simulink model "BODE"  (R2018b)
settings: Solver=VariableStepAuto  StartTime=0.0  StopTime=10.0  RelTol=1e-3
libraries: slctrlblks x1
settings Model: Creator=xpess  LastModifiedBy=xpess

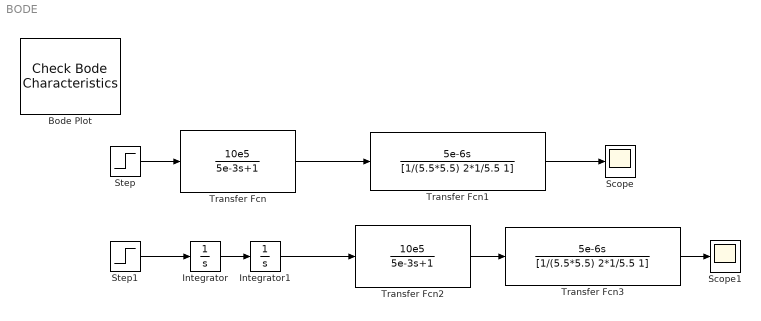
== system BODE ==
  Bode Plot : slctrlblks/Model Verification/Check Bode  Characteristics  InstantiateOnLoad=on  SaveOperatingPoints=off  LinearizationIOs={'/Step', 1, 'in', 'on', '';'/Transfer Fcn1', 1, 'out', 'on', ''}  LinearizeAt=SnapshotTimes  SnapshotTimes=[0]  TriggerType=rising  SampleTime=auto  RateConversionMethod=zoh  PreWarpFreq=10  UseExactDelayModel=off  UseFullBlockNameLabels=off  UseBusSignalLabels=off  enabled=on  stopWhenAssertionFail=off  export=off  ViewDlgPos=[412.333333333333 81 510 390]  OpenViewOnLoad=off  LaunchViewOnOpen=on  FrequencyUnits=rad/s  MagnitudeUnits=dB  PhaseUnits=deg  TimeUnits=seconds  EnableUpperBound=off  UpperBoundFrequencies=[]  UpperBoundMagnitudes=[]  EnableLowerBound=off  LowerBoundFrequencies=[]  LowerBoundMagnitudes=[]
      settings: SourceProductName=Simulink Control Design
  Integrator : Integrator
  Integrator1 : Integrator
  Scope : Scope
  Scope1 : Scope
  Step : Step  Time=0  SampleTime=0
  Step1 : Step  Time=0  SampleTime=0
  Transfer Fcn : TransferFcn  Numerator=[10e5]  Denominator=[5e-3 1]
  Transfer Fcn1 : TransferFcn  Numerator=[5e-6 0]  Denominator=[1/(5.5*5.5) 2*1/5.5 1]
  Transfer Fcn2 : TransferFcn  Numerator=[10e5]  Denominator=[5e-3 1]
  Transfer Fcn3 : TransferFcn  Numerator=[5e-6 0]  Denominator=[1/(5.5*5.5) 2*1/5.5 1]
  wires:
  Transfer Fcn/1 -> Transfer Fcn1/1
  Step/1 -> Transfer Fcn/1
  Transfer Fcn1/1 -> Scope/1
  Step1/1 -> Integrator/1
  Transfer Fcn2/1 -> Transfer Fcn3/1
  Transfer Fcn3/1 -> Scope1/1
  Integrator/1 -> Integrator1/1
  Integrator1/1 -> Transfer Fcn2/1
